simulink model "LinkFDR"  (R2014b)
settings: Solver=ode45  StartTime=0.0  StopTime=10.0  RelTol=1e-3
values from neighbouring files (symbols this model uses):
  DH_c = obj.Data.DH_Child    [Link.m]    (also in OpenKinematicChain.m = obj.Parameters.Kinematics.DH_c; OpenKinematicChainExample.m = [        pi/2    d1      a1      pi/2; OpenKinemticChainExample.m = [        pi/2    d1      a1      pi/2; SerialManipulatorExample.m = [        pi/2    d1      a1      pi/2)
  DH_p = obj.Data.DH_Parent    [Link.m]    (also in OpenKinematicChain.m = obj.Parameters.Kinematics.DH_p; OpenKinematicChainExample.m = [        0       0       0       0; OpenKinemticChainExample.m = [        0       0       0       0; SerialManipulator.m = zeros(N,4))
  I = obj.Dynamics.I    [LinkData.m]    (also in OpenKinematicChain.m = obj.Parameters.Dynamics.I; OpenKinematicChainExample.m = cat(3,cat(3,cat(3,I1,I2),I3),I4); OpenKinemticChainExample.m = cat(3,cat(3,cat(3,I1,I2),I3),I4); SerialManipulatorExample.m = cat(3,cat(3,I1,I2),I3))
  m = obj.Dynamics.m    [LinkData.m]    (also in OpenKinematicChain.m = obj.Parameters.Dynamics.m; OpenKinematicChainExample.m = [m1;m2;m3;m4]; OpenKinemticChainExample.m = [m1;m2;m3;m4]; SerialManipulatorExample.m = [m1;m2;m3])
  N = obj.DOF    [OpenKinematicChain.m]    (also in OpenKinematicChainExample.m = numel(rho); OpenKinemticChainExample.m = numel(rho); SerialManipulator.m = numel(rho); SerialManipulatorExample.m = numel(rho))
  s = obj.Relative_Pose.p    [Frame.m]    (also in Point.m = obj.Relative_Position)
undefined symbols (not defined in the file or in its folder): X, Y, Z
undefined symbols (not defined in the file): cm, q, qd
libraries: sm_lib x12, nesl_utility x4
settings Model: Creator=tchoopojcharoen  LastModifiedBy=tchoopojcharoen

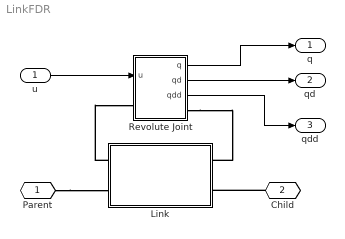
== system LinkFDR ==
  u : Inport
  Link : Subsystem  mask{DH_p=DH_p, DH_c=DH_c, m=m, cm=cm, I=I}
      mask prompts: DH_p "DH_Parent"; DH_c "DH_Child"; m "Mass"; cm "Center of Mass"; I "Inertia"
  Revolute Joint : Subsystem  mask{q=q, qd=qd}
  Parent : PMIOPort  Port=1  Side=Left
  Child : PMIOPort  Port=2  Side=Right
  q : Outport
  qd : Outport  Port=2
  qdd : Outport  Port=3
  wires:
  Revolute Joint/2(qd) -> qd/1
  Revolute Joint/1(q) -> q/1
  Revolute Joint/3(qdd) -> qdd/1
  u/1 -> Revolute Joint/1(u)
  connections:
  Link/LConn1 -- Revolute Joint/LConn1
  Revolute Joint/RConn1 -- Link/RConn1
  Parent/RConn1 -- Link/LConn2
  Child/RConn1 -- Link/RConn2

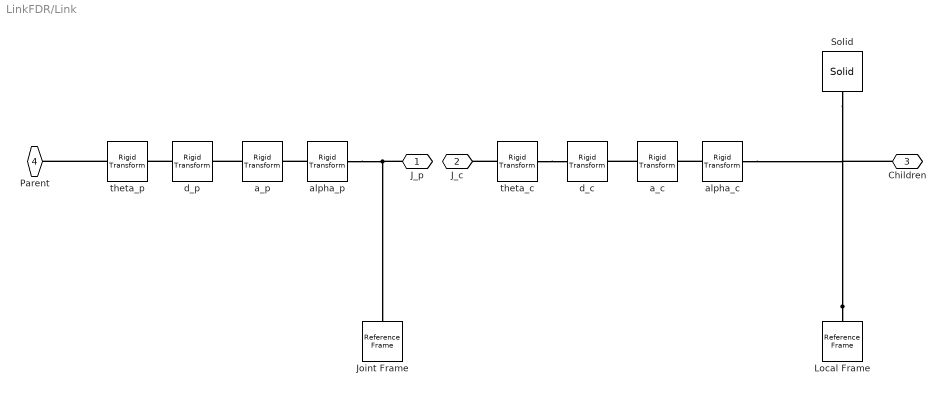
== system LinkFDR/Link ==
  Joint Frame : sm_lib/Frames and Transforms/Reference Frame  BlockFunction=simmechanics.library.frames_transforms.reference_frame
  Local Frame : sm_lib/Frames and Transforms/Reference Frame  BlockFunction=simmechanics.library.frames_transforms.reference_frame
  Solid : sm_lib/Body Elements/Solid  InertiaType=Custom  Mass=m  MassUnits=kg  CenterOfMass=cm'  CenterOfMassUnits=m  MomentsOfInertia=[I(1,1) I(2,2) I(3,3)]  MomentsOfInertiaUnits=kg*m^2  ProductsOfInertia=[I(1,2) I(1,3) I(2,3)]  ProductsOfInertiaUnits=kg*m^2  DensityBased=on  Density=1000  DensityUnits=kg/(m^3)  GraphicType=None  MarkerShape=Sphere  MarkerSize=10  MarkerSizeUnits=m  GraphicVisPropType=SimpleVisualProperties  GraphicDiffuseColor=[0.5 0.5 0.5]  GraphicSpecularColor=[0.5 0.5 0.5 1.0]  GraphicAmbientColor=[0.15 0.15 0.15 1.0]  GraphicEmissiveColor=[0.0 0.0 0.0 1.0]  GraphicShininess=75  GraphicOpacity=1.0  GeometryShape=Brick  RectangleSize=[1 1]  RectangleSizeUnits=m  BrickDimensions=[1 1 1]  BrickDimensionUnits=m  CylinderRadius=1  CylinderRadiusUnits=m  CylinderLength=1  CylinderLengthUnits=m  SphereRadius=1  SphereRadiusUnits=m  EllipsoidRadii=[1 1 1]  EllipsoidRadiiUnits=m  ExtrusionCrossSection=[1 1; -1 1; -1 -1; 1 -1]  ExtrusionCrossSectionUnits=m  ExtrusionLength=1  ExtrusionLengthUnits=m  PolygonNumSides=3  PolygonOuterRadius=1  PolygonOuterRadiusUnits=m  ExtGeomFileType=STL  ExtGeomFileUnits=m  RevolutionCrossSection=[1 1; 1 -1; 2 -1; 2 1]  RevolutionCrossSectionUnits=m  RevolutionExtent=Full  RevolutionAngle=180  RevolutionAngleUnits=deg  BlockFunction=simmechanics.library.body_elements.solid
  a_c : sm_lib/Frames and Transforms/Rigid Transform  TranslationMethod=StandardAxis  TranslationLengthUnit=m  TranslationStandardAxis=+X  TranslationStandardOffset=DH_c(3)  TranslationCartesianOffset=[0 0 0]  TranslationROffset=0  TranslationROffsetUnits=m  TranslationZOffset=0  TranslationZOffsetUnits=m  TranslationThetaOffset=0  TranslationThetaOffsetUnits=deg  RotationMethod=None  RotationAngleUnits=deg  RotationStandardAxis=+Z  RotationAngle=0.0  RotationArbitraryAxis=[0 0 1]  FollAlignAxisA=+X  BaseAlignAxisA=+Y  FollAlignAxisB=+Y  BaseAlignAxisB=+Z  RotationMatrix=[1 0 0; 0 1 0; 0 0 1]  BlockFunction=simmechanics.library.frames_transforms.rigid_transform
  a_p : sm_lib/Frames and Transforms/Rigid Transform  TranslationMethod=StandardAxis  TranslationLengthUnit=m  TranslationStandardAxis=+X  TranslationStandardOffset=DH_p(3)  TranslationCartesianOffset=[0 0 0]  TranslationROffset=0  TranslationROffsetUnits=m  TranslationZOffset=0  TranslationZOffsetUnits=m  TranslationThetaOffset=0  TranslationThetaOffsetUnits=deg  RotationMethod=None  RotationAngleUnits=deg  RotationStandardAxis=+Z  RotationAngle=0.0  RotationArbitraryAxis=[0 0 1]  FollAlignAxisA=+X  BaseAlignAxisA=+Y  FollAlignAxisB=+Y  BaseAlignAxisB=+Z  RotationMatrix=[1 0 0; 0 1 0; 0 0 1]  BlockFunction=simmechanics.library.frames_transforms.rigid_transform
  alpha_c : sm_lib/Frames and Transforms/Rigid Transform  TranslationMethod=None  TranslationLengthUnit=m  TranslationStandardAxis=+X  TranslationStandardOffset=DH_p(4)  TranslationCartesianOffset=[0 0 0]  TranslationROffset=0  TranslationROffsetUnits=m  TranslationZOffset=0  TranslationZOffsetUnits=m  TranslationThetaOffset=0  TranslationThetaOffsetUnits=deg  RotationMethod=StandardAxis  RotationAngleUnits=rad  RotationStandardAxis=+X  RotationAngle=DH_c(4)  RotationArbitraryAxis=[0 0 1]  FollAlignAxisA=+X  BaseAlignAxisA=+Y  FollAlignAxisB=+Y  BaseAlignAxisB=+Z  RotationMatrix=[1 0 0; 0 1 0; 0 0 1]  BlockFunction=simmechanics.library.frames_transforms.rigid_transform
  alpha_p : sm_lib/Frames and Transforms/Rigid Transform  TranslationMethod=None  TranslationLengthUnit=m  TranslationStandardAxis=+X  TranslationStandardOffset=DH_p(4)  TranslationCartesianOffset=[0 0 0]  TranslationROffset=0  TranslationROffsetUnits=m  TranslationZOffset=0  TranslationZOffsetUnits=m  TranslationThetaOffset=0  TranslationThetaOffsetUnits=deg  RotationMethod=StandardAxis  RotationAngleUnits=rad  RotationStandardAxis=+X  RotationAngle=DH_p(4)  RotationArbitraryAxis=[0 0 1]  FollAlignAxisA=+X  BaseAlignAxisA=+Y  FollAlignAxisB=+Y  BaseAlignAxisB=+Z  RotationMatrix=[1 0 0; 0 1 0; 0 0 1]  BlockFunction=simmechanics.library.frames_transforms.rigid_transform
  d_c : sm_lib/Frames and Transforms/Rigid Transform  TranslationMethod=StandardAxis  TranslationLengthUnit=m  TranslationStandardAxis=+Z  TranslationStandardOffset=DH_c(2)  TranslationCartesianOffset=[0 0 0]  TranslationROffset=0  TranslationROffsetUnits=m  TranslationZOffset=0  TranslationZOffsetUnits=m  TranslationThetaOffset=0  TranslationThetaOffsetUnits=deg  RotationMethod=None  RotationAngleUnits=deg  RotationStandardAxis=+Z  RotationAngle=0.0  RotationArbitraryAxis=[0 0 1]  FollAlignAxisA=+X  BaseAlignAxisA=+Y  FollAlignAxisB=+Y  BaseAlignAxisB=+Z  RotationMatrix=[1 0 0; 0 1 0; 0 0 1]  BlockFunction=simmechanics.library.frames_transforms.rigid_transform
  d_p : sm_lib/Frames and Transforms/Rigid Transform  TranslationMethod=StandardAxis  TranslationLengthUnit=m  TranslationStandardAxis=+Z  TranslationStandardOffset=DH_p(2)  TranslationCartesianOffset=[0 0 0]  TranslationROffset=0  TranslationROffsetUnits=m  TranslationZOffset=0  TranslationZOffsetUnits=m  TranslationThetaOffset=0  TranslationThetaOffsetUnits=deg  RotationMethod=None  RotationAngleUnits=deg  RotationStandardAxis=+Z  RotationAngle=0.0  RotationArbitraryAxis=[0 0 1]  FollAlignAxisA=+X  BaseAlignAxisA=+Y  FollAlignAxisB=+Y  BaseAlignAxisB=+Z  RotationMatrix=[1 0 0; 0 1 0; 0 0 1]  BlockFunction=simmechanics.library.frames_transforms.rigid_transform
  theta_c : sm_lib/Frames and Transforms/Rigid Transform  TranslationMethod=None  TranslationLengthUnit=m  TranslationStandardAxis=+Z  TranslationStandardOffset=DH_c(2)  TranslationCartesianOffset=[0 0 0]  TranslationROffset=0  TranslationROffsetUnits=m  TranslationZOffset=0  TranslationZOffsetUnits=m  TranslationThetaOffset=0  TranslationThetaOffsetUnits=deg  RotationMethod=StandardAxis  RotationAngleUnits=rad  RotationStandardAxis=+Z  RotationAngle=DH_c(1)  RotationArbitraryAxis=[0 0 1]  FollAlignAxisA=+X  BaseAlignAxisA=+Y  FollAlignAxisB=+Y  BaseAlignAxisB=+Z  RotationMatrix=[1 0 0; 0 1 0; 0 0 1]  BlockFunction=simmechanics.library.frames_transforms.rigid_transform
  theta_p : sm_lib/Frames and Transforms/Rigid Transform  TranslationMethod=None  TranslationLengthUnit=m  TranslationStandardAxis=+Z  TranslationStandardOffset=0  TranslationCartesianOffset=[0 0 0]  TranslationROffset=0  TranslationROffsetUnits=m  TranslationZOffset=0  TranslationZOffsetUnits=m  TranslationThetaOffset=0  TranslationThetaOffsetUnits=deg  RotationMethod=StandardAxis  RotationAngleUnits=rad  RotationStandardAxis=+Z  RotationAngle=DH_p(1)  RotationArbitraryAxis=[0 0 1]  FollAlignAxisA=+X  BaseAlignAxisA=+Y  FollAlignAxisB=+Y  BaseAlignAxisB=+Z  RotationMatrix=[1 0 0; 0 1 0; 0 0 1]  BlockFunction=simmechanics.library.frames_transforms.rigid_transform
  J_p : PMIOPort  Port=1  Side=Left
  J_c : PMIOPort  Port=2  Side=Right
  Children : PMIOPort  Port=3  Side=Right
  Parent : PMIOPort  Port=4  Side=Left
  connections:
  a_p/LConn1 -- d_p/RConn1
  Local Frame/RConn1 -- alpha_c/RConn1 -- Solid/RConn1 -- Children/RConn1
  theta_p/LConn1 -- Parent/RConn1
  theta_c/RConn1 -- d_c/LConn1
  alpha_p/RConn1 -- J_p/RConn1 -- Joint Frame/RConn1
  alpha_p/LConn1 -- a_p/RConn1
  d_p/LConn1 -- theta_p/RConn1
  alpha_c/LConn1 -- a_c/RConn1
  a_c/LConn1 -- d_c/RConn1
  theta_c/LConn1 -- J_c/RConn1

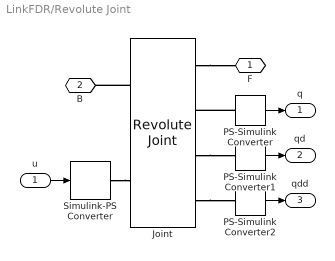
== system LinkFDR/Revolute Joint ==
  u : Inport
  Joint : sm_lib/Joints/Revolute Joint  SenseConstraintForce=off  SenseConstraintForceX=off  SenseConstraintForceY=off  SenseConstraintForceZ=off  SenseConstraintTorque=off  SenseConstraintTorqueX=off  SenseConstraintTorqueY=off  SenseConstraintTorqueZ=off  SenseTotalForce=off  SenseTotalForceX=off  SenseTotalForceY=off  SenseTotalForceZ=off  SenseTotalTorque=off  SenseTotalTorqueX=off  SenseTotalTorqueY=off  SenseTotalTorqueZ=off  CompositeWrenchDir=FollowerOnBase  CompositeWrenchFrame=BaseFrame  EquilibriumPosition=0  EquilibriumPositionUnits=deg  SpringStiffness=0  SpringStiffnessUnits=N*m/deg  DampingCoefficient=0  DampingCoefficientUnits=N*m/(deg/s)  TorqueActuationMode=InputTorque  MotionActuationMode=ComputedMotion  SensePosition=on  SenseVelocity=on  SenseAcceleration=on  SenseTorqueForce=off  PositionTargetValue=q  PositionTargetValueUnits=rad  PositionTargetSpecify=on  PositionTargetPriority=High  VelocityTargetValue=qd  VelocityTargetValueUnits=rad/s  VelocityTargetSpecify=on  VelocityTargetPriority=High  BlockFunction=simmechanics.library.joints.revolute_joint
  PS-Simulink Converter : nesl_utility/PS-Simulink Converter  PhysicalDomain=network_engine_domain  SubClassName=ps_output  LeftPortType=input  RightPortType=output  PseudoPeriodic=off  Frequencies=[]  Unit=1  AffineConversion=off
  PS-Simulink Converter1 : nesl_utility/PS-Simulink Converter  PhysicalDomain=network_engine_domain  SubClassName=ps_output  LeftPortType=input  RightPortType=output  PseudoPeriodic=off  Frequencies=[]  Unit=1  AffineConversion=off
  PS-Simulink Converter2 : nesl_utility/PS-Simulink Converter  PhysicalDomain=network_engine_domain  SubClassName=ps_output  LeftPortType=input  RightPortType=output  PseudoPeriodic=off  Frequencies=[]  Unit=1  AffineConversion=off
  Simulink-PS Converter : nesl_utility/Simulink-PS Converter  PhysicalDomain=network_engine_domain  SubClassName=ps_input  LeftPortType=input  RightPortType=output  PseudoPeriodic=off  Frequencies=[]  NoiseDistribution=none  NoiseParameters=[]  Unit=1  AffineConversion=off  InputFiltering=off  SimscapeFilterOrder=1  InputFilterTimeConstant=0.001  UdotUserProvided=2
  F : PMIOPort  Port=1  Side=Right
  B : PMIOPort  Port=2  Side=Left
  q : Outport
  qd : Outport  Port=2
  qdd : Outport  Port=3
  wires:
  PS-Simulink Converter/1 -> q/1
  u/1 -> Simulink-PS Converter/1
  PS-Simulink Converter1/1 -> qd/1
  PS-Simulink Converter2/1 -> qdd/1
  connections:
  Simulink-PS Converter/RConn1 -- Joint/LConn2
  Joint/LConn1 -- B/RConn1
  Joint/RConn1 -- F/RConn1
  PS-Simulink Converter/LConn1 -- Joint/RConn2
  Joint/RConn3 -- PS-Simulink Converter1/LConn1
  Joint/RConn4 -- PS-Simulink Converter2/LConn1
